simulink model "StreetLaneSegment"  (R2021a)
settings: Solver=VariableStepAuto  StartTime=0.0  StopTime=10.0  RelTol=1e-3
settings Model: Creator=phill  LastModifiedBy=phill

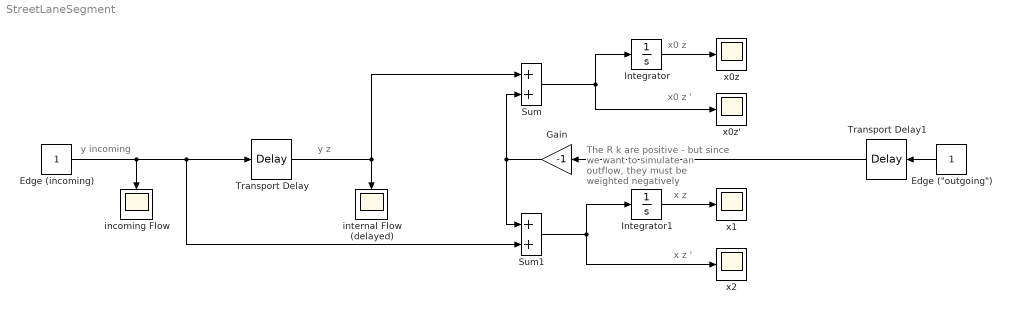
== system StreetLaneSegment ==
  note: The R k are positive - but since we
      | want to simulate an outflow, they
      | must be weighted negatively
  note: y incoming
  note: y z
  note: x0 z
  note: x0 z '
  note: x z
  note: x z '
  "Edge (\"outgoing\")" : Constant
  Edge (incoming) : Constant
  Gain : Gain  Gain=-1
  Integrator : Integrator
  Integrator1 : Integrator
  Sum : Sum
  Sum1 : Sum
  Transport Delay : TransportDelay  DelayTime=3
  Transport Delay1 : TransportDelay  DelayTime=6
  incoming Flow : Scope
  internal Flow (delayed) : Scope
  x0z : Scope
  x0z' : Scope
  x1 : Scope
  x2 : Scope
  wires:
  Edge (incoming)/1 -> Sum1/2, Transport Delay/1, incoming Flow/1
  Transport Delay/1 -> internal Flow (delayed)/1, Sum/1
  Transport Delay1/1 -> Gain/1
  Sum/1 -> x0z'/1, Integrator/1
  Integrator/1 -> x0z/1
  Integrator1/1 -> x1/1
  Sum1/1 -> x2/1, Integrator1/1
  "Edge (\"outgoing\")"/1 -> Transport Delay1/1
  Gain/1 -> Sum1/1, Sum/2
